simulink model "Drone_Simulation"  (R2020a)
settings: Solver=ode1  StartTime=0.0  StopTime=50  FixedStep=1e-3
values from neighbouring files (symbols this model uses):
  AeEMSC = 1    [Qball_X8_Model.m]
  alpha1TDDBSC = 1    [Qball_X8_Model.m]    (also in ReliabilityModel_Script.m = 0.7)
  bBNG = 1.2    [ReliabilityModel_Script.m]
  bEMSC = 1    [Qball_X8_Model.m]
  bEVCAP = 1    [Qball_X8_Model.m]    (also in ReliabilityModel_Script.m = 1.1)
  BNG_Motor1 = 0.8    [ReliabilityModel_Script.m]
  BNG_Motor2 = 1    [ReliabilityModel_Script.m]
  BNG_Motor3 = 1    [ReliabilityModel_Script.m]
  BNG_Motor4 = 1    [ReliabilityModel_Script.m]
  BNG_Motor5 = 1    [ReliabilityModel_Script.m]
  BNG_Motor6 = 1    [ReliabilityModel_Script.m]
  bp = 0.001    [ControlLawsScript.m]    (also in ControlLaws_Script.m)
  bq = 0.001    [ControlLawsScript.m]    (also in ControlLaws_Script.m)
  br = 0.001    [ControlLawsScript.m]    (also in ControlLaws_Script.m)
  bTDDBSC = 1    [Qball_X8_Model.m]    (also in ReliabilityModel_Script.m = 1.1)
  bWDG = 1    [Qball_X8_Model.m]    (also in ReliabilityModel_Script.m = 1.1)
  C_A = [     k_T           k_T          k_T                k_T          k_T         k_T ... (first row only)    [ControlLawsScript.m]    (also in ControlLaws_Script.m)
  C_mot = 1    [Qball_X8_Model.m]    (also in ReliabilityModel_Script.m = 17.46)
  C_th_esc = 1    [Qball_X8_Model.m]    (also in ReliabilityModel_Script.m = 1.67)
  CAPEV_Motor1 = 0.8    [ReliabilityModel_Script.m]
  CAPEV_Motor2 = 1    [ReliabilityModel_Script.m]
  CAPEV_Motor3 = 1    [ReliabilityModel_Script.m]
  CAPEV_Motor4 = 1    [ReliabilityModel_Script.m]
  CAPEV_Motor5 = 1    [ReliabilityModel_Script.m]
  CAPEV_Motor6 = 1    [ReliabilityModel_Script.m]
  cdx = cx*m    (= 17.4057414746)    [ControlLawsScript.m]    (also in ControlLaws_Script.m)
  cdy = cy*m    (= 17.4057414746)    [ControlLawsScript.m]    (also in ControlLaws_Script.m)
  cdz = cz*m    (= 17.4057414746)    [ControlLawsScript.m]    (also in ControlLaws_Script.m)
  EaEMSC = 1    [Qball_X8_Model.m]
  EaEVCAP = 1    [Qball_X8_Model.m]    (also in ReliabilityModel_Script.m = 0.94)
  EalphaTDDBSC = 1    [Qball_X8_Model.m]    (also in ReliabilityModel_Script.m = 0.7)
  EaTDDBSC = 1    [Qball_X8_Model.m]    (also in ReliabilityModel_Script.m = 0.7)
  EaWDG = 1    [Qball_X8_Model.m]    (also in ReliabilityModel_Script.m = 0.5)
  g = 9.80665    [ControlLawsScript.m]    (also in ControlLaws_Script.m; Qball_X8_Model.m = 9.87)
  JrefEMSC = 1    [Qball_X8_Model.m]
  Jz = 0.15887270137511    (= 0.158872701375)    [ControlLawsScript.m]    (also in ControlLaws_Script.m)
  k_b = 1    [Qball_X8_Model.m]    (also in ReliabilityModel_Script.m = -21.8546)
  Kp = (Jx/Tc)-bp    (= 4.11390529802)    [ControlLawsScript.m]    (also in ControlLaws_Script.m)
  Kp2 = Jx*((4/ts))*((-4/ts)+((bp+Kp)/Jx))/Kp    (= 6.72163348437)    [ControlLawsScript.m]    (also in ControlLaws_Script.m)
  Kq = (Jy/Tc)-bq    (= 4.12186008142)    [ControlLawsScript.m]    (also in ControlLaws_Script.m)
  Kq2 = Jy*((4/ts))*((-4/ts)+((bq+Kq)/Jy))/Kq    (= 6.72163033191)    [ControlLawsScript.m]    (also in ControlLaws_Script.m)
  Kr = (Jz/(tsy/25))-br    (= 7.94263506876)    [ControlLawsScript.m]    (also in ControlLaws_Script.m)
  Kr2 = Jz*((4/tsy))*((-4/tsy)+((br+Kr)/Jz))/Kr    (= 6.72084606682)    [ControlLawsScript.m]    (also in ControlLaws_Script.m)
  kv = 1/930    (= 0.0010752688172)    [StingerScript.m]
  Kx = abs(Kx)    [ControlLawsScript.m]    (also in ControlLaws_Script.m)
  Ky = abs(Ky)    [ControlLawsScript.m]    (also in ControlLaws_Script.m)
  Kz = (m/Tcz)-cz    (= 38.5143536865)    [ControlLawsScript.m]    (also in ControlLaws_Script.m)
  Kz2 = m*((4/tsz))*((-4/tsz)+((cz+Kz)/m))/Kz    (= 1.89810050529)    [ControlLawsScript.m]    (also in ControlLaws_Script.m)
  LnomEMSC = 1    [Qball_X8_Model.m]
  LnomEVCAP = 1    [Qball_X8_Model.m]    (also in ReliabilityModel_Script.m = 10800000)
  LnomTDDBSC = 1    [Qball_X8_Model.m]    (also in ReliabilityModel_Script.m = 9997200)
  LnomWDG = 1    [Qball_X8_Model.m]    (also in ReliabilityModel_Script.m = 72000000)
  m = 3.4811482949175    (= 3.48114829492)    [ControlLawsScript.m]    (also in ControlLaws_Script.m; Qball_X8_Model.m = 1.45)
  max_yaw_moment = k_y*hov_thrust/k_T    (= 0.323744079512)    [ControlLawsScript.m]    (also in ControlLaws_Script.m = 0.57666914163)
  NEMSC = 1    [Qball_X8_Model.m]
  nEVCAP = 1    [Qball_X8_Model.m]    (also in ReliabilityModel_Script.m)
  pconst = 2    [Qball_X8_Model.m]    (also in ReliabilityModel_Script.m)
  pitch_angle_limit = 32/R2D    (= 0.558505360638)    [ControlLawsScript.m]    (also in ControlLaws_Script.m)
  R2D = 180/pi    (= 57.2957795131)    [ControlLawsScript.m]    (also in ControlLaws_Script.m)
  R_th_esc = 1    [Qball_X8_Model.m]    (also in ReliabilityModel_Script.m = 5.14)
  R_th_mot = 1    [Qball_X8_Model.m]    (also in ReliabilityModel_Script.m = 8.59)
  Re = 0.008    [Qball_X8_Model.m]    (also in ReliabilityModel_Script.m)
  roll_angle_limit = 32/R2D    (= 0.558505360638)    [ControlLawsScript.m]    (also in ControlLaws_Script.m)
  RrefBNG = 0.9    [ReliabilityModel_Script.m]
  RrefEMSC = 1    [Qball_X8_Model.m]
  RrefEVCAP = 1    [Qball_X8_Model.m]    (also in ReliabilityModel_Script.m = 0.9)
  RrefTDDBSC = 1    [Qball_X8_Model.m]    (also in ReliabilityModel_Script.m = 0.37)
  RrefWDG = 1    [Qball_X8_Model.m]    (also in ReliabilityModel_Script.m = 0.98)
  SCTDDB_Motor1 = 0.8    [ReliabilityModel_Script.m]
  SCTDDB_Motor2 = 1    [ReliabilityModel_Script.m]
  SCTDDB_Motor3 = 1    [ReliabilityModel_Script.m]
  SCTDDB_Motor4 = 1    [ReliabilityModel_Script.m]
  SCTDDB_Motor5 = 1    [ReliabilityModel_Script.m]
  SCTDDB_Motor6 = 1    [ReliabilityModel_Script.m]
  T_amb = 1    [Qball_X8_Model.m]    (also in ReliabilityModel_Script.m = 20)
  T_amb_mot = 1    [Qball_X8_Model.m]    (also in ReliabilityModel_Script.m = 20)
  t_D_SCTDDB = 30    [ReliabilityModel_Script.m]
  TrefEMSC = 1    [Qball_X8_Model.m]
  TrefEVCAP = 1    [Qball_X8_Model.m]    (also in ReliabilityModel_Script.m = 105)
  TrefTDDBSC = 1    [Qball_X8_Model.m]    (also in ReliabilityModel_Script.m = 150)
  TrefWDG = 1    [Qball_X8_Model.m]    (also in ReliabilityModel_Script.m = 40)
  Ub = 12    [Qball_X8_Model.m]    (also in ReliabilityModel_Script.m)
  VmaxEVCAP = 1    [Qball_X8_Model.m]    (also in ReliabilityModel_Script.m = 35)
  VnomEVCAP = 1    [Qball_X8_Model.m]    (also in ReliabilityModel_Script.m = 35)
  WDG_Motor1 = 0.8    [ReliabilityModel_Script.m]
  WDG_Motor2 = 1    [ReliabilityModel_Script.m]
  WDG_Motor3 = 1    [ReliabilityModel_Script.m]
  WDG_Motor4 = 1    [ReliabilityModel_Script.m]
  WDG_Motor5 = 1    [ReliabilityModel_Script.m]
  WDG_Motor6 = 1    [ReliabilityModel_Script.m]
  z_x = cx    (= 5)    [ControlLawsScript.m]    (also in ControlLaws_Script.m)
  z_y = cy    (= 5)    [ControlLawsScript.m]    (also in ControlLaws_Script.m)
undefined symbols (not defined in the file or in its folder): FuselageContactForces, LeftAftArm, LeftAftSkid, LeftArm, LeftFrontArm, LeftFrontSkid, LeftSideContactForces, Lower, missionPlanX, missionPlanY, missionPlanYaw, missionPlanZ, Newton, Raphson, RightAftArm, RightAftSkid, RightArm, RightFrontArm, RightFrontSkid, RightSideContactForces, SkidsContactForces, timeConstant, Upper, X, Y, Z
libraries: sm_lib x90, nesl_utility x78, fl_lib x61, ee_lib x19, dspinverses x1, dspmtrx3 x1
(part 3 of 5)

== system Drone_Simulation/CONTROL ALLOCATION/Reliability Observer (SCEM)/LambdaEM ==
  In1 : Inport
  In2 : Inport  Port=2
  Bias : Bias  Bias=-1
  Divide : Product  Inputs=*/
  Divide1 : Product  Inputs=**/
  Math Function : Math  Operator=pow  SaturateOnIntegerOverflow=on
  bEMSC : Constant  Value=bEMSC
  Out1 : Outport
  wires:
  Math Function/1 -> Divide1/1
  bEMSC/1 -> Bias/1, Divide1/2
  Divide/1 -> Math Function/1
  Bias/1 -> Math Function/2
  In2/1 -> Divide1/3, Divide/2
  In1/1 -> Divide/1
  Divide1/1 -> Out1/1

== system Drone_Simulation/CONTROL ALLOCATION/Reliability Observer (SCTDDB)1/Cumulative Aging VTDDB ==
  T_IN : Inport
  V_ESC_OUT : Inport  Port=2
  Aging Velocity1 : Product
  Cumulative Aging1 : Integrator  InitialConditionSource=external
  Display{,1..3} (4 alike) : Display
  Divide : Product  Inputs=**
  Divide1 : Product  Inputs=*/
  Divide2 : Product  Inputs=/*/
  Divide3 : Product  Inputs=**//
  EaTDDBSC : Constant  Value=EaTDDBSC
  Gain : Gain  Gain=-1
  Gain1 : Gain  Gain=-1
  K : Constant  Value=k_b  VectorParams1D=off
  Math Function1 : Math  SaturateOnIntegerOverflow=on
  Math Function2 : Math  SaturateOnIntegerOverflow=on
  Motors Reliability Initial Condition : Constant  Value=[SCTDDB_Motor1,SCTDDB_Motor2,SCTDDB_Motor3,SCTDDB_Motor4,SCTDDB_Motor5,SCTDDB_Motor6]
  alpha1TDDBSC : Constant  Value=alpha1TDDBSC
  t_D_SCTDDB : Constant  Value=t_D_SCTDDB
  Out1 : Outport
  wires:
  Divide/1 -> Display/1, Cumulative Aging1/2
  [VrefTDDB] -> Divide/2, Display3/1
  Motors Reliability Initial Condition/1 -> Divide/1
  T_IN/1 -> Divide3/4, Display1/1, Divide2/1
  Aging Velocity1/1 -> Cumulative Aging1/1
  V_ESC_OUT/1 -> Divide1/1
  Divide3/1 -> Math Function2/1
  Divide1/1 -> Gain/1
  t_D_SCTDDB/1 -> Divide1/2
  Cumulative Aging1/1 -> Out1/1
  Divide2/1 -> Math Function1/1
  Math Function2/1 -> Aging Velocity1/2
  EaTDDBSC/1 -> Gain1/1
  K/1 -> Divide2/3, Divide3/3
  Math Function1/1 -> Aging Velocity1/1
  alpha1TDDBSC/1 -> Divide3/1
  Gain/1 -> Divide3/2, Display2/1
  Gain1/1 -> Divide2/2

== system Drone_Simulation/CONTROL ALLOCATION/Reliability Observer (SCTDDB)1/LambdaTDDB ==
  In1 : Inport
  In2 : Inport  Port=2
  Bias : Bias  Bias=-1
  Divide : Product  Inputs=*/
  Divide1 : Product  Inputs=**/
  Math Function : Math  Operator=pow  SaturateOnIntegerOverflow=on
  bTDDBSC : Constant  Value=bTDDBSC
  Out1 : Outport
  wires:
  In1/1 -> Divide/1
  In2/1 -> Divide/2, Divide1/3
  Divide/1 -> Math Function/1
  Math Function/1 -> Divide1/1
  bTDDBSC/1 -> Bias/1, Divide1/2
  Bias/1 -> Math Function/2
  Divide1/1 -> Out1/1

== system Drone_Simulation/CONTROL ALLOCATION/Reliability Observer (SCTDDB)1/ReliabilityTDDB ==
  In1 : Inport
  In2 : Inport  Port=2
  Abs : Abs
  Divide2 : Product  Inputs=*//
  Math Function1 : Math  Operator=reciprocal  SaturateOnIntegerOverflow=on
  Math Function2 : Math  Operator=pow  SaturateOnIntegerOverflow=on
  Math Function3 : Math  Operator=pow  SaturateOnIntegerOverflow=on
  Math Function4 : Math  Operator=log  SaturateOnIntegerOverflow=on
  R(V) : Math  SaturateOnIntegerOverflow=on
  RrefTDDBSC : Constant  Value=RrefTDDBSC
  Unary Minus : UnaryMinus
  Unary Minus1 : UnaryMinus
  bTDDBSC1 : Constant  Value=bTDDBSC
  Out1 : Outport
  wires:
  In1/1 -> Divide2/1
  Divide2/1 -> Math Function3/1
  Abs/1 -> Math Function2/1
  Math Function3/1 -> Unary Minus1/1
  Math Function2/1 -> Divide2/3
  In2/1 -> Divide2/2
  Math Function4/1 -> Abs/1
  RrefTDDBSC/1 -> Math Function4/1
  Math Function1/1 -> Math Function2/2
  Unary Minus1/1 -> R(V)/1
  bTDDBSC1/1 -> Unary Minus/1, Math Function3/2
  Unary Minus/1 -> Math Function1/1
  R(V)/1 -> Out1/1

== system Drone_Simulation/CONTROL ALLOCATION/Reliability Observer (SCTDDB)1/VrefTDDB ==
  Display : Display
  Divide4 : Product  Inputs=/*/
  Divide5 : Product  Inputs=**//
  EaTDDBSC1 : Constant  Value=EaTDDBSC
  EalphaTDDBSC : Constant  Value=EalphaTDDBSC
  K1 : Constant  Value=k_b  VectorParams1D=off
  LnomTDDBSC : Constant  Value=LnomTDDBSC
  Math Function3 : Math  SaturateOnIntegerOverflow=on
  Math Function4 : Math  SaturateOnIntegerOverflow=on
  TrefTDDBSC1 : Constant  Value=TrefTDDBSC
  Unary Minus2 : UnaryMinus
  Unary Minus3 : UnaryMinus
  Vref : Product  Inputs=3
  alpha1TDDBSC1 : Constant  Value=alpha1TDDBSC
  Out1 : Outport
  tag scope: VrefTDDB=global
  wires:
  Vref/1 -> Out1/1, [VrefTDDB]
  Divide4/1 -> Math Function3/1
  Divide5/1 -> Math Function4/1, Display/1
  Math Function4/1 -> Vref/2
  Math Function3/1 -> Vref/1
  Unary Minus2/1 -> Divide4/2
  EaTDDBSC1/1 -> Unary Minus2/1
  Unary Minus3/1 -> Divide5/2
  LnomTDDBSC/1 -> Vref/3
  TrefTDDBSC1/1 -> Divide4/1, Divide5/4
  alpha1TDDBSC1/1 -> Divide5/1
  EalphaTDDBSC/1 -> Unary Minus3/1
  K1/1 -> Divide5/3, Divide4/3

== system Drone_Simulation/CONTROL ALLOCATION/Reliability Observer (WDG)1/Cumulative Aging WDG ==
  In1 : Inport
  Cumulative Aging : Integrator  InitialConditionSource=external
  Display{,1..6} (7 alike) : Display
  Divide : Product  Inputs=**
  Divide2 : Product  Inputs=/*/
  EaWDG : Constant  Value=EaWDG
  Gain : Gain  Gain=10000
  K : Constant  Value=k_b
  Math Function1 : Math  SaturateOnIntegerOverflow=on
  Motors Reliability Initial Condition : Constant  Value=[WDG_Motor1,WDG_Motor2,WDG_Motor3,WDG_Motor4,WDG_Motor5,WDG_Motor6]
  Unary Minus : UnaryMinus
  Out1 : Outport
  wires:
  Gain/1 -> Divide/2, Display1/1
  Divide/1 -> Display/1, Cumulative Aging/2
  Motors Reliability Initial Condition/1 -> Divide/1, Display2/1
  [VrefWDG] -> Gain/1
  In1/1 -> Divide2/1, Display4/1
  Unary Minus/1 -> Divide2/2
  Divide2/1 -> Math Function1/1
  K/1 -> Divide2/3, Display6/1
  EaWDG/1 -> Unary Minus/1, Display5/1
  Math Function1/1 -> Cumulative Aging/1, Display3/1
  Cumulative Aging/1 -> Out1/1

== system Drone_Simulation/CONTROL ALLOCATION/Reliability Observer (WDG)1/Lambda ==
  In1 : Inport
  In2 : Inport  Port=2
  Bias : Bias  Bias=-1
  Divide : Product  Inputs=*/
  Divide1 : Product  Inputs=**/
  Math Function : Math  Operator=pow  SaturateOnIntegerOverflow=on
  bWDG1 : Constant  Value=bWDG
  Out1 : Outport
  wires:
  In1/1 -> Divide/1
  Divide/1 -> Math Function/1
  bWDG1/1 -> Bias/1, Divide1/2
  In2/1 -> Divide/2, Divide1/3
  Divide1/1 -> Out1/1
  Math Function/1 -> Divide1/1
  Bias/1 -> Math Function/2

== system Drone_Simulation/CONTROL ALLOCATION/Reliability Observer (WDG)1/ReliabilityWDG ==
  In1 : Inport
  In2 : Inport  Port=2
  Abs : Abs
  Divide3 : Product  Inputs=*//
  Math Function2 : Math  Operator=pow  SaturateOnIntegerOverflow=on
  Math Function3 : Math  Operator=pow  SaturateOnIntegerOverflow=on
  Math Function4 : Math  Operator=log  SaturateOnIntegerOverflow=on
  Math Function5 : Math  Operator=reciprocal  SaturateOnIntegerOverflow=on
  R(V) : Math  SaturateOnIntegerOverflow=on
  RrefWDG : Constant  Value=RrefWDG
  Unary Minus1 : UnaryMinus
  Unary Minus2 : UnaryMinus
  bWDG : Constant  Value=bWDG
  Out1 : Outport
  wires:
  In1/1 -> Divide3/1
  Unary Minus2/1 -> Math Function5/1
  Math Function2/1 -> Divide3/3
  RrefWDG/1 -> Math Function4/1
  Math Function5/1 -> Math Function2/2
  Math Function3/1 -> Unary Minus1/1
  bWDG/1 -> Unary Minus2/1, Math Function3/2
  In2/1 -> Divide3/2
  R(V)/1 -> Out1/1
  Unary Minus1/1 -> R(V)/1
  Math Function4/1 -> Abs/1
  Abs/1 -> Math Function2/1
  Divide3/1 -> Math Function3/1

== system Drone_Simulation/CONTROL ALLOCATION/Reliability Observer (WDG)1/VrefWDG ==
  Display{,1..5} (6 alike) : Display
  Divide4 : Product  Inputs=/*/
  EaWDG1 : Constant  Value=EaWDG
  K1 : Constant  Value=k_b
  LnomWDG : Constant  Value=LnomWDG
  Math Function6 : Math  SaturateOnIntegerOverflow=on
  TrefWDG : Constant  Value=TrefWDG
  Unary Minus3 : UnaryMinus
  Vref : Product
  Out1 : Outport
  tag scope: VrefWDG=global
  wires:
  Vref/1 -> Out1/1
  TrefWDG/1 -> Display4/1, Divide4/1, [VrefWDG]
  Divide4/1 -> Math Function6/1, Display2/1
  Math Function6/1 -> Vref/2, Display1/1
  LnomWDG/1 -> Vref/1, Display/1
  K1/1 -> Display3/1, Divide4/3
  Unary Minus3/1 -> Divide4/2, Display5/1
  EaWDG1/1 -> Unary Minus3/1

== system Drone_Simulation/PLANT MODEL/BODY/SKIDS ==
  Left Skid : sm_lib/Body Elements/File Solid  ExtGeomFileName=STL files\Skids.stl  UnitType=Custom  ExtGeomFileUnits=mm  StepReaderType=HEX  ExportConvexHullGeometry=off  InertiaType=CalculateFromGeometry  Mass=1  MassUnits=kg  CenterOfMass=[0 0 0]  CenterOfMassUnits=m  MomentsOfInertia=[1 1 1]  MomentsOfInertiaUnits=kg*m^2  ProductsOfInertia=[0 0 0]  ProductsOfInertiaUnits=kg*m^2  BasedOnType=Density  Density=rho2  DensityUnits=kg/m^3  DoExposeReferenceFrame=on  SerializedFrames=<Frames/>  GraphicType=FromGeometry  MarkerShape=Sphere  MarkerSize=10  GraphicVisPropType=SimpleVisualProperties  GraphicDiffuseColor=rgb2  GraphicSpecularColor=[0.5 0.5 0.5 1.0]  GraphicAmbientColor=[0.15 0.15 0.15 1.0]  GraphicEmissiveColor=[0.0 0.0 0.0 1.0]  GraphicShininess=75  GraphicOpacity=op2
  Right Contact Skids : SimscapeBus  HierarchyStrings=LeftAftSkid;LeftFrontSkid;RightFrontSkid;RightAftSkid
  Right Skid : sm_lib/Body Elements/File Solid  ExtGeomFileName=STL files\Skids.stl  UnitType=Custom  ExtGeomFileUnits=mm  StepReaderType=HEX  ExportConvexHullGeometry=off  InertiaType=CalculateFromGeometry  Mass=1  MassUnits=kg  CenterOfMass=[0 0 0]  CenterOfMassUnits=m  MomentsOfInertia=[1 1 1]  MomentsOfInertiaUnits=kg*m^2  ProductsOfInertia=[0 0 0]  ProductsOfInertiaUnits=kg*m^2  BasedOnType=Density  Density=rho2  DensityUnits=kg/m^3  DoExposeReferenceFrame=on  SerializedFrames=<Frames/>  GraphicType=FromGeometry  MarkerShape=Sphere  MarkerSize=10  GraphicVisPropType=SimpleVisualProperties  GraphicDiffuseColor=rgb2  GraphicSpecularColor=[0.5 0.5 0.5 1.0]  GraphicAmbientColor=[0.15 0.15 0.15 1.0]  GraphicEmissiveColor=[0.0 0.0 0.0 1.0]  GraphicShininess=75  GraphicOpacity=op2
  Rigid Transform1 : sm_lib/Frames and Transforms/Rigid Transform  TranslationMethod=Cartesian  TranslationStandardOffset=0  TranslationLengthUnit=m  TranslationStandardAxis=+Z  TranslationCartesianOffset=[D/2+0.015 D/2-0.0415 -H/2-0.0925]  TranslationROffset=0  TranslationROffsetUnits=m  TranslationZOffset=0  TranslationZOffsetUnits=m  TranslationThetaOffset=0  TranslationThetaOffsetUnits=deg  RotationMethod=None  RotationAngleUnits=deg  RotationStandardAxis=+X  RotationAngle=180  RotationArbitraryAxis=[0 0 1]  FollAlignAxisA=+X  BaseAlignAxisA=+Y  FollAlignAxisB=+Y  BaseAlignAxisB=+Z  RotationSequenceAxes=FollowerAxes  RotationSequence=XYX  RotationSequenceAngles=[0 0 0]  RotationSequenceAnglesUnits=deg  RotationMatrix=[1 0 0; 0 1 0; 0 0 1]
  Rigid Transform2 : sm_lib/Frames and Transforms/Rigid Transform  TranslationMethod=Cartesian  TranslationStandardOffset=0  TranslationLengthUnit=m  TranslationStandardAxis=+Z  TranslationCartesianOffset=[D/2+0.015 -D/2+0.0415 -H/2-0.0925]  TranslationROffset=0  TranslationROffsetUnits=m  TranslationZOffset=0  TranslationZOffsetUnits=m  TranslationThetaOffset=0  TranslationThetaOffsetUnits=deg  RotationMethod=None  RotationAngleUnits=deg  RotationStandardAxis=+X  RotationAngle=180  RotationArbitraryAxis=[0 0 1]  FollAlignAxisA=+X  BaseAlignAxisA=+Y  FollAlignAxisB=+Y  BaseAlignAxisB=+Z  RotationSequenceAxes=FollowerAxes  RotationSequence=XZY  RotationSequenceAngles=[180 180 0]  RotationSequenceAnglesUnits=deg  RotationMatrix=[1 0 0; 0 1 0; 0 0 1]
  Rigid Transform3 : sm_lib/Frames and Transforms/Rigid Transform  TranslationMethod=Cartesian  TranslationStandardOffset=0  TranslationLengthUnit=m  TranslationStandardAxis=+Z  TranslationCartesianOffset=[-D/2-0.015 D/2-0.0415 -H/2-0.0925]  TranslationROffset=0  TranslationROffsetUnits=m  TranslationZOffset=0  TranslationZOffsetUnits=m  TranslationThetaOffset=0  TranslationThetaOffsetUnits=deg  RotationMethod=None  RotationAngleUnits=deg  RotationStandardAxis=+X  RotationAngle=180  RotationArbitraryAxis=[0 0 1]  FollAlignAxisA=+X  BaseAlignAxisA=+Y  FollAlignAxisB=+Y  BaseAlignAxisB=+Z  RotationSequenceAxes=FollowerAxes  RotationSequence=XYX  RotationSequenceAngles=[0 0 0]  RotationSequenceAnglesUnits=deg  RotationMatrix=[1 0 0; 0 1 0; 0 0 1]
  Rigid Transform4 : sm_lib/Frames and Transforms/Rigid Transform  TranslationMethod=Cartesian  TranslationStandardOffset=0  TranslationLengthUnit=m  TranslationStandardAxis=+Z  TranslationCartesianOffset=[-D/2-0.015 -D/2+0.0415 -H/2-0.0925]  TranslationROffset=0  TranslationROffsetUnits=m  TranslationZOffset=0  TranslationZOffsetUnits=m  TranslationThetaOffset=0  TranslationThetaOffsetUnits=deg  RotationMethod=None  RotationAngleUnits=deg  RotationStandardAxis=+X  RotationAngle=180  RotationArbitraryAxis=[0 0 1]  FollAlignAxisA=+X  BaseAlignAxisA=+Y  FollAlignAxisB=+Y  BaseAlignAxisB=+Z  RotationSequenceAxes=FollowerAxes  RotationSequence=XZY  RotationSequenceAngles=[180 180 0]  RotationSequenceAnglesUnits=deg  RotationMatrix=[1 0 0; 0 1 0; 0 0 1]
  Rigid Transform5 : sm_lib/Frames and Transforms/Rigid Transform  TranslationMethod=Cartesian  TranslationStandardOffset=0  TranslationLengthUnit=m  TranslationStandardAxis=+Z  TranslationCartesianOffset=[-0.188 D/2-0.032 -H/2]  TranslationROffset=0  TranslationROffsetUnits=m  TranslationZOffset=0  TranslationZOffsetUnits=m  TranslationThetaOffset=0  TranslationThetaOffsetUnits=deg  RotationMethod=StandardAxis  RotationAngleUnits=deg  RotationStandardAxis=+X  RotationAngle=180  RotationArbitraryAxis=[0 0 1]  FollAlignAxisA=+X  BaseAlignAxisA=+Y  FollAlignAxisB=+Y  BaseAlignAxisB=+Z  RotationSequenceAxes=FollowerAxes  RotationSequence=XYX  RotationSequenceAngles=[0 0 0]  RotationSequenceAnglesUnits=deg  RotationMatrix=[1 0 0; 0 1 0; 0 0 1]
  Rigid Transform6 : sm_lib/Frames and Transforms/Rigid Transform  TranslationMethod=Cartesian  TranslationStandardOffset=0  TranslationLengthUnit=m  TranslationStandardAxis=+Z  TranslationCartesianOffset=[0.188 -D/2+0.032 -H/2]  TranslationROffset=0  TranslationROffsetUnits=m  TranslationZOffset=0  TranslationZOffsetUnits=m  TranslationThetaOffset=0  TranslationThetaOffsetUnits=deg  RotationMethod=RotationSequence  RotationAngleUnits=deg  RotationStandardAxis=+X  RotationAngle=180  RotationArbitraryAxis=[0 0 1]  FollAlignAxisA=+X  BaseAlignAxisA=+Y  FollAlignAxisB=+Y  BaseAlignAxisB=+Z  RotationSequenceAxes=FollowerAxes  RotationSequence=XZY  RotationSequenceAngles=[180 180 0]  RotationSequenceAnglesUnits=deg  RotationMatrix=[1 0 0; 0 1 0; 0 0 1]
  Spherical Solid{,1..3} (4 alike) : sm_lib/Body Elements/Spherical Solid  GraphicAmbientColor=[0.15 0.15 0.15 1.0]  BasedOnType=Density  CenterOfMass=[0 0 0]  CenterOfMassUnits=m  GraphicDiffuseColor=rgb2  Density=0  DensityUnits=kg/m^3  DoExposeReferenceFrame=on  GraphicEmissiveColor=[0.0 0.0 0.0 1.0]  ExportEntireGeometry=on  SerializedExposedGeometries=<ExposedGeometries><ExposedGeometry><RawGeometryId>entire</RawGeometryId><ExposedGeometryId>G</ExposedGeometryId></ExposedGeometry></ExposedGeometries>  SerializedFrames=<Frames/>  MarkerShape=Sphere  MarkerSize=10  GraphicType=None  InertiaType=CalculateFromGeometry  Mass=1  MassUnits=kg  MomentsOfInertia=[1 1 1]  MomentsOfInertiaUnits=kg*m^2  GraphicOpacity=op2  ProductsOfInertia=[0 0 0]  ProductsOfInertiaUnits=kg*m^2  GraphicShininess=75  GraphicSpecularColor=[0.5 0.5 0.5 1.0]  SphereRadius=0.0095  SphereRadiusUnits=m  GraphicVisPropType=SimpleVisualProperties
  Contact : PMIOPort  Side=Left
  Fuselage : PMIOPort  Port=2  Side=Left
  connections:
  Contact/RConn1 -- Right Contact Skids/RConn1
  Left Skid/RConn1 -- Rigid Transform5/RConn1
  Rigid Transform6/RConn1 -- Right Skid/RConn1
  Spherical Solid/RConn1 -- Rigid Transform1/RConn1
  Rigid Transform2/RConn1 -- Spherical Solid1/RConn1
  Fuselage/RConn1 -- Rigid Transform4/LConn1 -- Rigid Transform2/LConn1 -- Rigid Transform3/LConn1 -- Rigid Transform1/LConn1 -- Rigid Transform5/LConn1 -- Rigid Transform6/LConn1
  Rigid Transform4/RConn1 -- Spherical Solid3/RConn1
  Rigid Transform3/RConn1 -- Spherical Solid2/RConn1
  Right Contact Skids/LConn2 -- Spherical Solid/LConn1
  Right Contact Skids/LConn3 -- Spherical Solid1/LConn1
  Right Contact Skids/LConn4 -- Spherical Solid3/LConn1
  Right Contact Skids/LConn1 -- Spherical Solid2/LConn1

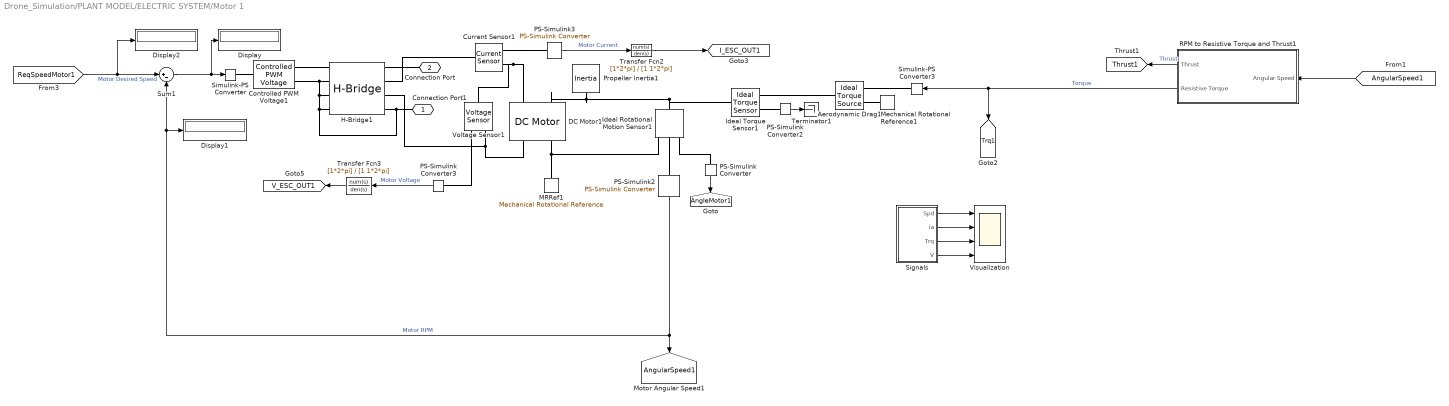
== system Drone_Simulation/PLANT MODEL/ELECTRIC SYSTEM/Motor 1 ==
  Aerodynamic Drag1 : fl_lib/Mechanical/Mechanical Sources/Ideal Torque Source
  Controlled PWM Voltage1 : ee_lib/Integrated Circuits/Controlled PWM Voltage  F=freq Hz  TD=0 s  pulse_width_offset=0 s  pulse_min=0 s  Vmin=0 V  Vmax=5 V  Vm=1 V  pwm_or_av=1  event_type=2  sample_time=Samp_time s  u_min=0  u_max=1
      settings: InternalSimscapePortConfiguration="{\"Bottom\":[],\"Left\":[{\"id\":\"u\",\"label\":\"u\",\"type\":\"input\"}],\"Right\":[{\"id\":\"p2\",\"label\":\"PWM\",\"type\":\"foundation.electrical.electrical\"},{\"id\":\"n2\",\"label\":\"REF\",\"type\":\"foundation.electrical.electrical\"}],\"Top\":[]}"
  Current Sensor1 : fl_lib/Electrical/Electrical Sensors/Current Sensor
  DC Motor1 : ee_lib/Electromechanical/Brushed Motors/DC Motor  field_option=ee.enum.field_option.pm  Rf=100 Ohm  Lf=1 H  Laf=0.15 H  If0=0 A  parameterization=ee.enum.dcparam_option.circuit_param  Ra=R Ohm  La=100 uH  emf_or_torque=ee.enum.emf_or_torque.kv  Kv=Kv V/rpm  Ki=kv N*m/A  T_stall=0.1 N*m  w_max=4000 rpm  w_rated=2500 rpm  P_rated=10 W  V_rated=12 V  J=0 kg*m^2  lam_param=ee.enum.lam_param.current  lam=0.5e-5 N*m/(rad/s)  i_noload=Ic A  V_i_noload=14.8 V  speed0=0 rpm  alpha=3.93e-3 1/K  Tmeas=25 degC  thermal_mass=100 J/K  initial_temperature=25 degC
  Display : Display
  Display1 : Display
  Display2 : Display
  H-Bridge1 : ee_lib/Semiconductors & Converters/Converters/H-Bridge  supply_ports=ee.enum.supply_ports.showsupply  Venable=0.01 V  Vmax=5 V  Vreverse=10000 V  Vbrake=10000 V  Vm=12 V  pwm_or_av=ee.enum.pwm_or_av.pwm  regenerative_braking_mode=ee.enum.converters.regenerative_braking_mode.always_enabled  discontinuous=ee.enum.current_profile.continuous  freewheeling_mode=ee.enum.converters.freewheeling_mode.two_switches_one_diode  Ron=0.00001 Ohm  Don=0.1 Ohm  Goff=1e-6 S  Rload=3.38+0.1 Ohm  Lload=1e-5 H  F=4 kHz  thermal_mass=100 J/K  initial_temperature=298.15 K  Ron2=0.1 Ohm  Don2=0.05 Ohm  Tmeas=298.15 K  Tmeas2=398.15 K
      settings: InternalSimscapePortConfiguration="{\"Bottom\":[],\"Left\":[{\"id\":\"ENA\",\"label\":\"PWM\",\"type\":\"foundation.electrical.electrical\"},{\"id\":\"REF\",\"label\":\"REF\",\"type\":\"foundation.electrical.electrical\"},{\"id\":\"REV\",\"label\":\"REV\",\"type\":\"foundation.electrical.electrical\"},{\"id\":\"BRK\",\"label\":\"BRK\",\"type\":\"foundation.electrical.electrical\"}],\"Right\":[{\"id\":\"p1\",\"label\":\"V+\",\"type\":\"foundation.electrical.electrical\"},{\"id\":\"p2\",\"label\":\"+\",\"type\":\"foundation.electrical.electrical\"},{\"id\":\"n2\",\"label\":\"-\",\"type\":\"foundation.electrical.electrical\"},{\"id\":\"n1\",\"label\":\"V-\",\"type\":\"foundation.electrical.electrical\"}],\"Top\":[]}"
  Ideal Rotational Motion Sensor1 : fl_lib/Mechanical/Mechanical Sensors/Ideal Rotational Motion Sensor  wrap_angle=simscape.enum.onoff.off  offset=0 deg
  Ideal Torque Sensor1 : fl_lib/Mechanical/Mechanical Sensors/Ideal Torque Sensor
  MRRef1 : fl_lib/Mechanical/Rotational Elements/Mechanical Rotational Reference
  Mechanical Rotational Reference1 : fl_lib/Mechanical/Rotational Elements/Mechanical Rotational Reference
  PS-Simulink Converter : nesl_utility/PS-Simulink Converter  PhysicalDomain=network_engine_domain  SubClassName=ps_output  LeftPortType=input  RightPortType=output  PseudoPeriodic=off  Frequencies=[]  Unit=inherit  AffineConversion=off
  PS-Simulink Converter2 : nesl_utility/PS-Simulink Converter  PhysicalDomain=network_engine_domain  SubClassName=ps_output  LeftPortType=input  RightPortType=output  PseudoPeriodic=off  Frequencies=[]  Unit=inherit  AffineConversion=off
  PS-Simulink Converter3 : nesl_utility/PS-Simulink Converter  PhysicalDomain=network_engine_domain  SubClassName=ps_output  LeftPortType=input  RightPortType=output  PseudoPeriodic=off  Frequencies=[]  Unit=inherit  AffineConversion=off
  PS-Simulink2 : nesl_utility/PS-Simulink Converter  PhysicalDomain=network_engine_domain  SubClassName=ps_output  LeftPortType=input  RightPortType=output  PseudoPeriodic=off  Frequencies=[]  Unit=rpm  AffineConversion=off
  PS-Simulink3 : nesl_utility/PS-Simulink Converter  PhysicalDomain=network_engine_domain  SubClassName=ps_output  LeftPortType=input  RightPortType=output  PseudoPeriodic=off  Frequencies=[]  Unit=A  AffineConversion=off
  Propeller Inertia1 : fl_lib/Mechanical/Rotational Elements/Inertia  inertia=J kg*m^2  w_specify=off  w_priority=High  w=0 rpm  w_nominal_specify=off  w_nominal_unit=rad/s  w_nominal_value=1  t_specify=off  t_priority=High  t=0 N*m  t_nominal_specify=off  t_nominal_unit=N*m  t_nominal_value=1
  RPM to Resistive Torque and Thrust1 : Subsystem
  Signals : Subsystem
  Simulink-PS Converter : nesl_utility/Simulink-PS Converter  PhysicalDomain=network_engine_domain  SubClassName=ps_input  LeftPortType=input  RightPortType=output  PseudoPeriodic=off  Frequencies=[]  NoiseDistribution=none  NoiseParameters=[]  Unit=1  AffineConversion=off  FilteringAndDerivatives=filter  SimscapeFilterOrder=1  InputFilterTimeConstant=0.001  UdotUserProvided=0
  Simulink-PS Converter3 : nesl_utility/Simulink-PS Converter  PhysicalDomain=network_engine_domain  SubClassName=ps_input  LeftPortType=input  RightPortType=output  PseudoPeriodic=off  Frequencies=[]  NoiseDistribution=none  NoiseParameters=[]  Unit=N*m  AffineConversion=off  FilteringAndDerivatives=provide  SimscapeFilterOrder=1  InputFilterTimeConstant=0.001  UdotUserProvided=0
  Sum1 : Sum  Inputs=|+-
  Terminator1 : Terminator
  Transfer Fcn2 : TransferFcn  Numerator=[1*2*pi]  Denominator=[1 1*2*pi]
  Transfer Fcn3 : TransferFcn  Numerator=[1*2*pi]  Denominator=[1 1*2*pi]
  Visualization : Scope  NumInputPorts=4
  Voltage Sensor1 : fl_lib/Electrical/Electrical Sensors/Voltage Sensor
  Connection Port1 : PMIOPort  Side=Left
  Connection Port : PMIOPort  Port=2  Side=Right
  tag scope: AngleMotor1=global, AngularSpeed1=global, I_ESC_OUT1=global, Thrust1=global, Trq1=global, V_ESC_OUT1=global
  wires:
  Signals/4(V) -> Visualization/4
  Signals/2(ia) -> Visualization/2
  Signals/3(Trq) -> Visualization/3
  Signals/1(Spd) -> Visualization/1
  RPM to Resistive Torque and Thrust1/2(Resistive Torque) -> [Trq1], Simulink-PS Converter3/1  "Torque"
  [ReqSpeedMotor1] -> Display2/1, Sum1/1  "Motor Desired Speed"
  PS-Simulink Converter2/1 -> Terminator1/1
  PS-Simulink2/1 -> Display1/1, Sum1/2, [AngularSpeed1]  "Motor RPM"
  RPM to Resistive Torque and Thrust1/1(Thrust) -> [Thrust1]  "Thrust"
  [AngularSpeed1] -> RPM to Resistive Torque and Thrust1/1(Angular Speed)
  Transfer Fcn2/1 -> [I_ESC_OUT1]
  PS-Simulink3/1 -> Transfer Fcn2/1  "Motor Current"
  Transfer Fcn3/1 -> [V_ESC_OUT1]
  PS-Simulink Converter3/1 -> Transfer Fcn3/1  "Motor Voltage"
  PS-Simulink Converter/1 -> [AngleMotor1]
  Sum1/1 -> Display/1, Simulink-PS Converter/1
  connections:
  Ideal Rotational Motion Sensor1/LConn1 -- Ideal Torque Sensor1/LConn1 -- DC Motor1/LConn2 -- Propeller Inertia1/LConn1
  Controlled PWM Voltage1/RConn2 -- H-Bridge1/LConn2 -- H-Bridge1/LConn3 -- H-Bridge1/RConn4 -- Connection Port1/RConn1 -- H-Bridge1/LConn4
  DC Motor1/RConn2 -- Ideal Rotational Motion Sensor1/RConn1 -- MRRef1/LConn1
  Ideal Rotational Motion Sensor1/RConn2 -- PS-Simulink2/LConn1
  Mechanical Rotational Reference1/LConn1 -- Aerodynamic Drag1/RConn2
  H-Bridge1/RConn3 -- DC Motor1/RConn1 -- Voltage Sensor1/RConn2
  H-Bridge1/LConn1 -- Controlled PWM Voltage1/RConn1
  PS-Simulink Converter2/LConn1 -- Ideal Torque Sensor1/RConn2
  Simulink-PS Converter3/RConn1 -- Aerodynamic Drag1/RConn1
  Ideal Torque Sensor1/RConn1 -- Aerodynamic Drag1/LConn1
  Current Sensor1/LConn1 -- H-Bridge1/RConn2
  Current Sensor1/RConn1 -- PS-Simulink3/LConn1
  DC Motor1/LConn1 -- Voltage Sensor1/LConn1 -- Current Sensor1/RConn2
  Voltage Sensor1/RConn1 -- PS-Simulink Converter3/LConn1
  Connection Port/RConn1 -- H-Bridge1/RConn1
  Simulink-PS Converter/RConn1 -- Controlled PWM Voltage1/LConn1
  PS-Simulink Converter/LConn1 -- Ideal Rotational Motion Sensor1/RConn3

== system Drone_Simulation/PLANT MODEL/ELECTRIC SYSTEM/Motor 2 ==
  Aerodynamic Drag : fl_lib/Mechanical/Mechanical Sources/Ideal Torque Source
  Controlled PWM Voltage : ee_lib/Integrated Circuits/Controlled PWM Voltage  F=freq Hz  TD=0 s  pulse_width_offset=0 s  pulse_min=0 s  Vmin=0 V  Vmax=5 V  Vm=1 V  pwm_or_av=1  event_type=2  sample_time=Samp_time s  u_min=0  u_max=1
      settings: InternalSimscapePortConfiguration="{\"Bottom\":[],\"Left\":[{\"id\":\"u\",\"label\":\"u\",\"type\":\"input\"}],\"Right\":[{\"id\":\"p2\",\"label\":\"PWM\",\"type\":\"foundation.electrical.electrical\"},{\"id\":\"n2\",\"label\":\"REF\",\"type\":\"foundation.electrical.electrical\"}],\"Top\":[]}"
  Current Sensor : fl_lib/Electrical/Electrical Sensors/Current Sensor
  DC Motor : ee_lib/Electromechanical/Brushed Motors/DC Motor  field_option=ee.enum.field_option.pm  Rf=100 Ohm  Lf=1 H  Laf=0.15 H  If0=0 A  parameterization=ee.enum.dcparam_option.circuit_param  Ra=R Ohm  La=100 uH  emf_or_torque=ee.enum.emf_or_torque.kv  Kv=Kv V/rpm  Ki=kv N*m/A  T_stall=0.1 N*m  w_max=4000 rpm  w_rated=2500 rpm  P_rated=10 W  V_rated=12 V  J=0 kg*m^2  lam_param=ee.enum.lam_param.current  lam=0.5e-5 N*m/(rad/s)  i_noload=Ic A  V_i_noload=14.8 V  speed0=0 rpm  alpha=3.93e-3 1/K  Tmeas=25 degC  thermal_mass=100 J/K  initial_temperature=25 degC
  H-Bridge : ee_lib/Semiconductors & Converters/Converters/H-Bridge  supply_ports=ee.enum.supply_ports.showsupply  Venable=0.01 V  Vmax=5 V  Vreverse=10000 V  Vbrake=10000 V  Vm=12 V  pwm_or_av=ee.enum.pwm_or_av.pwm  regenerative_braking_mode=ee.enum.converters.regenerative_braking_mode.always_enabled  discontinuous=ee.enum.current_profile.continuous  freewheeling_mode=ee.enum.converters.freewheeling_mode.two_switches_one_diode  Ron=0.00001 Ohm  Don=0.1 Ohm  Goff=1e-6 S  Rload=3.38+0.1 Ohm  Lload=1e-5 H  F=4 kHz  thermal_mass=100 J/K  initial_temperature=298.15 K  Ron2=0.1 Ohm  Don2=0.05 Ohm  Tmeas=298.15 K  Tmeas2=398.15 K
      settings: InternalSimscapePortConfiguration="{\"Bottom\":[],\"Left\":[{\"id\":\"ENA\",\"label\":\"PWM\",\"type\":\"foundation.electrical.electrical\"},{\"id\":\"REF\",\"label\":\"REF\",\"type\":\"foundation.electrical.electrical\"},{\"id\":\"REV\",\"label\":\"REV\",\"type\":\"foundation.electrical.electrical\"},{\"id\":\"BRK\",\"label\":\"BRK\",\"type\":\"foundation.electrical.electrical\"}],\"Right\":[{\"id\":\"p1\",\"label\":\"V+\",\"type\":\"foundation.electrical.electrical\"},{\"id\":\"p2\",\"label\":\"+\",\"type\":\"foundation.electrical.electrical\"},{\"id\":\"n2\",\"label\":\"-\",\"type\":\"foundation.electrical.electrical\"},{\"id\":\"n1\",\"label\":\"V-\",\"type\":\"foundation.electrical.electrical\"}],\"Top\":[]}"
  Ideal Rotational Motion Sensor : fl_lib/Mechanical/Mechanical Sensors/Ideal Rotational Motion Sensor  wrap_angle=simscape.enum.onoff.off  offset=0 deg
  Ideal Torque Sensor : fl_lib/Mechanical/Mechanical Sensors/Ideal Torque Sensor
  MRRef : fl_lib/Mechanical/Rotational Elements/Mechanical Rotational Reference
  Mechanical Rotational Reference2 : fl_lib/Mechanical/Rotational Elements/Mechanical Rotational Reference
  PS-Simulink : nesl_utility/PS-Simulink Converter  PhysicalDomain=network_engine_domain  SubClassName=ps_output  LeftPortType=input  RightPortType=output  PseudoPeriodic=off  Frequencies=[]  Unit=rpm  AffineConversion=off
  PS-Simulink Converter : nesl_utility/PS-Simulink Converter  PhysicalDomain=network_engine_domain  SubClassName=ps_output  LeftPortType=input  RightPortType=output  PseudoPeriodic=off  Frequencies=[]  Unit=inherit  AffineConversion=off
  PS-Simulink Converter1 : nesl_utility/PS-Simulink Converter  PhysicalDomain=network_engine_domain  SubClassName=ps_output  LeftPortType=input  RightPortType=output  PseudoPeriodic=off  Frequencies=[]  Unit=inherit  AffineConversion=off
  PS-Simulink Converter3 : nesl_utility/PS-Simulink Converter  PhysicalDomain=network_engine_domain  SubClassName=ps_output  LeftPortType=input  RightPortType=output  PseudoPeriodic=off  Frequencies=[]  Unit=inherit  AffineConversion=off
  PS-Simulink3 : nesl_utility/PS-Simulink Converter  PhysicalDomain=network_engine_domain  SubClassName=ps_output  LeftPortType=input  RightPortType=output  PseudoPeriodic=off  Frequencies=[]  Unit=A  AffineConversion=off
  Propeller Inertia : fl_lib/Mechanical/Rotational Elements/Inertia  inertia=J kg*m^2  w_specify=off  w_priority=High  w=0 rpm  w_nominal_specify=off  w_nominal_unit=rad/s  w_nominal_value=1  t_specify=off  t_priority=High  t=0 N*m  t_nominal_specify=off  t_nominal_unit=N*m  t_nominal_value=1
  RPM to Resistive Torque and Thrust : Subsystem
  Signals : Subsystem
  Simulink-PS Converter : nesl_utility/Simulink-PS Converter  PhysicalDomain=network_engine_domain  SubClassName=ps_input  LeftPortType=input  RightPortType=output  PseudoPeriodic=off  Frequencies=[]  NoiseDistribution=none  NoiseParameters=[]  Unit=1  AffineConversion=off  FilteringAndDerivatives=filter  SimscapeFilterOrder=1  InputFilterTimeConstant=0.001  UdotUserProvided=0
  Simulink-PS Converter1 : nesl_utility/Simulink-PS Converter  PhysicalDomain=network_engine_domain  SubClassName=ps_input  LeftPortType=input  RightPortType=output  PseudoPeriodic=off  Frequencies=[]  NoiseDistribution=none  NoiseParameters=[]  Unit=N*m  AffineConversion=off  FilteringAndDerivatives=provide  SimscapeFilterOrder=1  InputFilterTimeConstant=0.001  UdotUserProvided=0
  Sum : Sum  Inputs=|+-
  Terminator : Terminator
  Transfer Fcn2 : TransferFcn  Numerator=[1*2*pi]  Denominator=[1 1*2*pi]
  Transfer Fcn3 : TransferFcn  Numerator=[1*2*pi]  Denominator=[1 1*2*pi]
  Visualization : Scope  NumInputPorts=4
  Voltage Sensor1 : fl_lib/Electrical/Electrical Sensors/Voltage Sensor
  Connection Port : PMIOPort  Side=Left
  Connection Port1 : PMIOPort  Port=2  Side=Left
  tag scope: AngleMotor2=global, AngularSpeed2=global, I_ESC_OUT2=global, Thrust2=global, Trq2=global, V_ESC_OUT2=global
  wires:
  RPM to Resistive Torque and Thrust/2(Resistive Torque) -> [Trq2], Simulink-PS Converter1/1  "Torque"
  [AngularSpeed2] -> RPM to Resistive Torque and Thrust/1(Angular Speed)
  RPM to Resistive Torque and Thrust/1(Thrust) -> [Thrust2]  "Thrust"
  PS-Simulink Converter1/1 -> Terminator/1
  PS-Simulink/1 -> Sum/2, [AngularSpeed2]  "Motor RPM"
  [ReqSpeedMotor2] -> Sum/1  "Motor Desired Speed"
  Transfer Fcn2/1 -> [I_ESC_OUT2]
  PS-Simulink3/1 -> Transfer Fcn2/1  "Motor Current"
  PS-Simulink Converter3/1 -> Transfer Fcn3/1  "Motor Voltage"
  Transfer Fcn3/1 -> [V_ESC_OUT2]
  PS-Simulink Converter/1 -> [AngleMotor2]
  Sum/1 -> Simulink-PS Converter/1
  Signals/1(Spd) -> Visualization/1
  Signals/3(Trq) -> Visualization/3
  Signals/2(ia) -> Visualization/2
  Signals/4(V) -> Visualization/4
  connections:
  Ideal Rotational Motion Sensor/RConn2 -- PS-Simulink/LConn1
  PS-Simulink Converter1/LConn1 -- Ideal Torque Sensor/RConn2
  Ideal Torque Sensor/RConn1 -- Aerodynamic Drag/LConn1
  Simulink-PS Converter1/RConn1 -- Aerodynamic Drag/RConn1
  Mechanical Rotational Reference2/LConn1 -- Aerodynamic Drag/RConn2
  Ideal Torque Sensor/LConn1 -- DC Motor/LConn2 -- Propeller Inertia/LConn1 -- Ideal Rotational Motion Sensor/LConn1
  Ideal Rotational Motion Sensor/RConn1 -- MRRef/LConn1 -- DC Motor/RConn2
  H-Bridge/RConn4 -- Connection Port/RConn1 -- H-Bridge/LConn4 -- H-Bridge/LConn3 -- H-Bridge/LConn2 -- Controlled PWM Voltage/RConn2
  H-Bridge/LConn1 -- Controlled PWM Voltage/RConn1
  Simulink-PS Converter/RConn1 -- Controlled PWM Voltage/LConn1
  H-Bridge/RConn3 -- DC Motor/RConn1 -- Voltage Sensor1/RConn2
  H-Bridge/RConn1 -- Connection Port1/RConn1
  PS-Simulink3/LConn1 -- Current Sensor/RConn1
  Current Sensor/LConn1 -- H-Bridge/RConn2
  Current Sensor/RConn2 -- Voltage Sensor1/LConn1 -- DC Motor/LConn1
  Voltage Sensor1/RConn1 -- PS-Simulink Converter3/LConn1
  PS-Simulink Converter/LConn1 -- Ideal Rotational Motion Sensor/RConn3

== system Drone_Simulation/PLANT MODEL/ELECTRIC SYSTEM/Motor 3 ==
  Aerodynamic Drag : fl_lib/Mechanical/Mechanical Sources/Ideal Torque Source
  Controlled PWM Voltage : ee_lib/Integrated Circuits/Controlled PWM Voltage  F=freq Hz  TD=0 s  pulse_width_offset=0 s  pulse_min=0 s  Vmin=0 V  Vmax=5 V  Vm=1 V  pwm_or_av=1  event_type=2  sample_time=Samp_time s  u_min=0  u_max=1
      settings: InternalSimscapePortConfiguration="{\"Bottom\":[],\"Left\":[{\"id\":\"u\",\"label\":\"u\",\"type\":\"input\"}],\"Right\":[{\"id\":\"p2\",\"label\":\"PWM\",\"type\":\"foundation.electrical.electrical\"},{\"id\":\"n2\",\"label\":\"REF\",\"type\":\"foundation.electrical.electrical\"}],\"Top\":[]}"
  Current Sensor : fl_lib/Electrical/Electrical Sensors/Current Sensor
  DC Motor : ee_lib/Electromechanical/Brushed Motors/DC Motor  field_option=ee.enum.field_option.pm  Rf=100 Ohm  Lf=1 H  Laf=0.15 H  If0=0 A  parameterization=ee.enum.dcparam_option.circuit_param  Ra=R Ohm  La=100 uH  emf_or_torque=ee.enum.emf_or_torque.kv  Kv=Kv V/rpm  Ki=kv N*m/A  T_stall=0.1 N*m  w_max=4000 rpm  w_rated=2500 rpm  P_rated=10 W  V_rated=12 V  J=0 kg*m^2  lam_param=ee.enum.lam_param.current  lam=0.5e-5 N*m/(rad/s)  i_noload=Ic A  V_i_noload=14.8 V  speed0=0 rpm  alpha=3.93e-3 1/K  Tmeas=25 degC  thermal_mass=100 J/K  initial_temperature=25 degC
  H-Bridge : ee_lib/Semiconductors & Converters/Converters/H-Bridge  supply_ports=ee.enum.supply_ports.showsupply  Venable=0.01 V  Vmax=5 V  Vreverse=10000 V  Vbrake=10000 V  Vm=12 V  pwm_or_av=ee.enum.pwm_or_av.pwm  regenerative_braking_mode=ee.enum.converters.regenerative_braking_mode.always_enabled  discontinuous=ee.enum.current_profile.continuous  freewheeling_mode=ee.enum.converters.freewheeling_mode.two_switches_one_diode  Ron=0.00001 Ohm  Don=0.1 Ohm  Goff=1e-6 S  Rload=3.38+0.1 Ohm  Lload=1e-5 H  F=4 kHz  thermal_mass=100 J/K  initial_temperature=298.15 K  Ron2=0.1 Ohm  Don2=0.05 Ohm  Tmeas=298.15 K  Tmeas2=398.15 K
      settings: InternalSimscapePortConfiguration="{\"Bottom\":[],\"Left\":[{\"id\":\"ENA\",\"label\":\"PWM\",\"type\":\"foundation.electrical.electrical\"},{\"id\":\"REF\",\"label\":\"REF\",\"type\":\"foundation.electrical.electrical\"},{\"id\":\"REV\",\"label\":\"REV\",\"type\":\"foundation.electrical.electrical\"},{\"id\":\"BRK\",\"label\":\"BRK\",\"type\":\"foundation.electrical.electrical\"}],\"Right\":[{\"id\":\"p1\",\"label\":\"V+\",\"type\":\"foundation.electrical.electrical\"},{\"id\":\"p2\",\"label\":\"+\",\"type\":\"foundation.electrical.electrical\"},{\"id\":\"n2\",\"label\":\"-\",\"type\":\"foundation.electrical.electrical\"},{\"id\":\"n1\",\"label\":\"V-\",\"type\":\"foundation.electrical.electrical\"}],\"Top\":[]}"
  Ideal Rotational Motion Sensor : fl_lib/Mechanical/Mechanical Sensors/Ideal Rotational Motion Sensor  wrap_angle=simscape.enum.onoff.off  offset=0 deg
  Ideal Torque Sensor : fl_lib/Mechanical/Mechanical Sensors/Ideal Torque Sensor
  MRRef : fl_lib/Mechanical/Rotational Elements/Mechanical Rotational Reference
  Mechanical Rotational Reference2 : fl_lib/Mechanical/Rotational Elements/Mechanical Rotational Reference
  PS-Simulink : nesl_utility/PS-Simulink Converter  PhysicalDomain=network_engine_domain  SubClassName=ps_output  LeftPortType=input  RightPortType=output  PseudoPeriodic=off  Frequencies=[]  Unit=rpm  AffineConversion=off
  PS-Simulink Converter : nesl_utility/PS-Simulink Converter  PhysicalDomain=network_engine_domain  SubClassName=ps_output  LeftPortType=input  RightPortType=output  PseudoPeriodic=off  Frequencies=[]  Unit=inherit  AffineConversion=off
  PS-Simulink Converter1 : nesl_utility/PS-Simulink Converter  PhysicalDomain=network_engine_domain  SubClassName=ps_output  LeftPortType=input  RightPortType=output  PseudoPeriodic=off  Frequencies=[]  Unit=inherit  AffineConversion=off
  PS-Simulink Converter3 : nesl_utility/PS-Simulink Converter  PhysicalDomain=network_engine_domain  SubClassName=ps_output  LeftPortType=input  RightPortType=output  PseudoPeriodic=off  Frequencies=[]  Unit=inherit  AffineConversion=off
  PS-Simulink3 : nesl_utility/PS-Simulink Converter  PhysicalDomain=network_engine_domain  SubClassName=ps_output  LeftPortType=input  RightPortType=output  PseudoPeriodic=off  Frequencies=[]  Unit=A  AffineConversion=off
  Propeller Inertia : fl_lib/Mechanical/Rotational Elements/Inertia  inertia=J kg*m^2  w_specify=off  w_priority=High  w=0 rpm  w_nominal_specify=off  w_nominal_unit=rad/s  w_nominal_value=1  t_specify=off  t_priority=High  t=0 N*m  t_nominal_specify=off  t_nominal_unit=N*m  t_nominal_value=1
  RPM to Resistive Torque and Thrust : Subsystem
  Signals : Subsystem
  Simulink-PS Converter : nesl_utility/Simulink-PS Converter  PhysicalDomain=network_engine_domain  SubClassName=ps_input  LeftPortType=input  RightPortType=output  PseudoPeriodic=off  Frequencies=[]  NoiseDistribution=none  NoiseParameters=[]  Unit=1  AffineConversion=off  FilteringAndDerivatives=filter  SimscapeFilterOrder=1  InputFilterTimeConstant=0.001  UdotUserProvided=0
  Simulink-PS Converter1 : nesl_utility/Simulink-PS Converter  PhysicalDomain=network_engine_domain  SubClassName=ps_input  LeftPortType=input  RightPortType=output  PseudoPeriodic=off  Frequencies=[]  NoiseDistribution=none  NoiseParameters=[]  Unit=N*m  AffineConversion=off  FilteringAndDerivatives=provide  SimscapeFilterOrder=1  InputFilterTimeConstant=0.001  UdotUserProvided=0
  Sum : Sum  Inputs=|+-
  Terminator : Terminator
  Transfer Fcn2 : TransferFcn  Numerator=[1*2*pi]  Denominator=[1 1*2*pi]
  Transfer Fcn3 : TransferFcn  Numerator=[1*2*pi]  Denominator=[1 1*2*pi]
  Visualization : Scope  NumInputPorts=4
  Voltage Sensor1 : fl_lib/Electrical/Electrical Sensors/Voltage Sensor
  Connection Port : PMIOPort  Side=Left
  Connection Port1 : PMIOPort  Port=2  Side=Right
  tag scope: AngleMotor3=global, AngularSpeed3=global, I_ESC_OUT3=global, Thrust3=global, Trq3=global, V_ESC_OUT3=global
  wires:
  RPM to Resistive Torque and Thrust/2(Resistive Torque) -> Simulink-PS Converter1/1, [Trq3]  "Torque"
  [AngularSpeed3] -> RPM to Resistive Torque and Thrust/1(Angular Speed)
  RPM to Resistive Torque and Thrust/1(Thrust) -> [Thrust3]
  PS-Simulink Converter1/1 -> Terminator/1
  PS-Simulink/1 -> Sum/2, [AngularSpeed3]  "Motor actual RPM"
  [ReqSpeedMotor3] -> Sum/1
  Transfer Fcn2/1 -> [I_ESC_OUT3]
  PS-Simulink3/1 -> Transfer Fcn2/1  "Motor Current"
  PS-Simulink Converter3/1 -> Transfer Fcn3/1  "Motor Voltage"
  Transfer Fcn3/1 -> [V_ESC_OUT3]
  PS-Simulink Converter/1 -> [AngleMotor3]
  Sum/1 -> Simulink-PS Converter/1
  Signals/4(V) -> Visualization/4
  Signals/3(Trq) -> Visualization/3
  Signals/2(ia) -> Visualization/2
  Signals/1(Spd) -> Visualization/1
  connections:
  Ideal Rotational Motion Sensor/RConn2 -- PS-Simulink/LConn1
  PS-Simulink Converter1/LConn1 -- Ideal Torque Sensor/RConn2
  Ideal Torque Sensor/RConn1 -- Aerodynamic Drag/LConn1
  Simulink-PS Converter1/RConn1 -- Aerodynamic Drag/RConn1
  Mechanical Rotational Reference2/LConn1 -- Aerodynamic Drag/RConn2
  Ideal Torque Sensor/LConn1 -- DC Motor/LConn2 -- Propeller Inertia/LConn1 -- Ideal Rotational Motion Sensor/LConn1
  Ideal Rotational Motion Sensor/RConn1 -- MRRef/LConn1 -- DC Motor/RConn2
  H-Bridge/LConn4 -- H-Bridge/RConn4 -- Connection Port/RConn1 -- H-Bridge/LConn3 -- Controlled PWM Voltage/RConn2 -- H-Bridge/LConn2
  Controlled PWM Voltage/RConn1 -- H-Bridge/LConn1
  Simulink-PS Converter/RConn1 -- Controlled PWM Voltage/LConn1
  DC Motor/RConn1 -- Voltage Sensor1/RConn2 -- H-Bridge/RConn3
  Connection Port1/RConn1 -- H-Bridge/RConn1
  Current Sensor/LConn1 -- Voltage Sensor1/LConn1 -- H-Bridge/RConn2
  PS-Simulink3/LConn1 -- Current Sensor/RConn1
  Current Sensor/RConn2 -- DC Motor/LConn1
  Voltage Sensor1/RConn1 -- PS-Simulink Converter3/LConn1
  PS-Simulink Converter/LConn1 -- Ideal Rotational Motion Sensor/RConn3
